simulink library "guidanceLawPathFollowingController"  (R2020a)
settings: Solver=VariableStepAuto  StartTime=0.0  StopTime=10.0  RelTol=1e-3
undefined symbols (not defined in the file or in its folder): env, initializeBussesFromBlock, maxRoll, vhcl
libraries: calculate_vector_magnitude x4, calcFluidDynamicLoads x1, eulAng2RotMat_ul x1, setpointToOutput_cl x1, alphaBeta_ul x1, calc_path_coordinates x1, ctrlAllocMatrix_cl x1, filteredPIDController_ul x1, findClosestPointOnPath x1, findTargetPathParameter x1, gnd2TanRotation_ul x1, spoolingController_cl x1
settings Model: Creator=Ayaz  LastModifiedBy=Ayaz

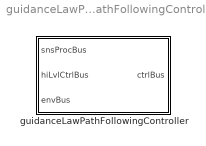
== system guidanceLawPathFollowingController ==
  guidanceLawPathFollowingController : Subsystem  LoadFcn=initializeBussesFromBlock(gcb)  InitFcn=initializeBussesFromBlock(gcb)  StartFcn=initializeBussesFromBlock(gcb)  mask{pathCtrl=90, vcl=vhcl, en=env}
      mask prompts: pathCtrl "Controller object"; vcl "Vehicle object"; en "Environment object"
      mask DialogControl ParameterGroupVar Prompt: Controller parameters
      mask DialogControl Container3 Prompt: Vehicle parameters
      mask DialogControl Container4 Prompt: Environment parameter

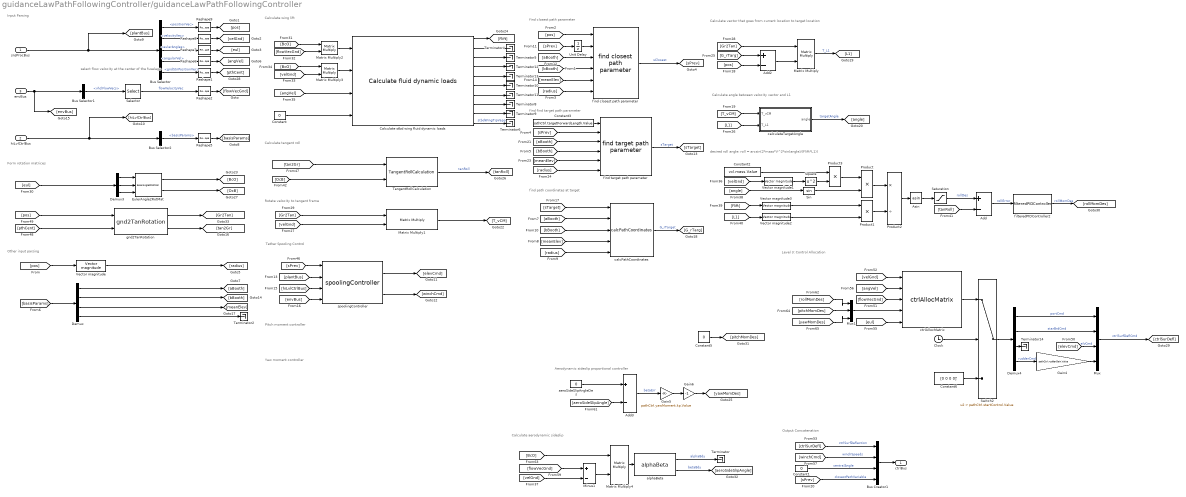
== system guidanceLawPathFollowingController/guidanceLawPathFollowingController ==
  note: Other input parsing
  note: Form rotation matrices
  note: Calculate wing lift
  note: Rotate velocity to tangent frame
  note: select flow velocity at the center of the fuselage
  note: Tether Spooling Control
  note: Input Parsing
  note: find closest path parameter
  note: find find target path parameter
  note: find path coordinates at target
  note: Calculate vector that goes from current location to target location
  note: Calculate angle between velocity vector and L1
  note: desired roll angle: roll = arcsin(2*mass*V^2*sin(angle)/(Flift*L1))
  note: Calculate tangent roll
  note: Output Concatenation
  note: Level 3: Control Allocation
  note: Pitch moment controller
  note: Aerodynamic sideslip proportional controller
  note: Yaw moment controller
  note: Calculate aerodynamic sideslip
  snsProcBus : Inport  OutDataTypeStr=Bus: sensorsProcessingBus
  hiLvlCtrlBus : Inport  Port=2  OutDataTypeStr=Bus: hiLvlCtrlBus
  envBus : Inport  Port=3  OutDataTypeStr=Bus: envBus
  Add : Sum  Inputs=+-
  Add2 : Sum  Inputs=+-
  Add3 : Sum  Inputs=+-
  Asin : Trigonometry  Operator=asin
  Bus Creator1 : BusCreator  Inputs=4  OutDataTypeStr=Bus: fltCtrlBus
      settings: InheritFromInputs=off
  Bus Selector : BusSelector  OutputSignals=positionVec,velocityVec,eulerAngles,angularVel,gndStnPositionVec
  Bus Selector1 : BusSelector  OutputSignals=vhclFlowVecs
  Bus Selector2 : BusSelector  OutputSignals=basisParams
  Calculate stbd wing fluid dynamic loads : calcFluidDynamicLoads/Calculate fluid dynamic loads  aSurf=vcl.stbdWing  sRef=vhcl.fluidRefArea.Value  rArm_LE=vcl.fluidMomentArms.Value(:,1).*[1;0;1]  rTip_LE=[0;0;0]  fluidDensity=en.water.density.Value
  Clock : Clock
  Constant : Constant  Value=0
  Constant1 : Constant  Value=0
  Constant2 : Constant  Value=vcl.mass.Value  VectorParams1D=off
  Constant3 : Constant  Value=pathCtrl.targetForwardLength.Value  VectorParams1D=off
  Constant5 : Constant  Value=0
  Constant6 : Constant  Value=[0 0 0 0]'
  Demux : Demux
  Demux3 : Demux  Outputs=3
  Demux4 : Demux
  EulerAngle2RotMat : eulAng2RotMat_ul/EulerAngle2RotMat  SystemSampleTime=-1  Latency=0  AutoFrameSizeCalculation=off
  Gain4 : Gain  Gain=pathCtrl.rudderGain.Value
  Gain5 : Gain  Gain=pathCtrl.yawMoment.kp.Value
  Gain6 : Gain  Gain=-1
  Matrix Multiply{,1..4} (5 alike) : Product  Multiplication=Matrix(*)
  Minus1 : Sum  Inputs=+-
  Mux : Mux
  Mux1 : Mux  Inputs=3
  Product : Product
  Product1 : Product
  Product2 : Product  Inputs=*/
  Product3 : Product
  Reshape{1..2,5..9} (7 alike) : Reshape  OutputDimensionality=Column vector (2-D)
  Saturation : Saturate  UpperLimit=maxRoll*pi/180  LowerLimit=-maxRoll*pi/180
  Selector : Selector  NumberOfDimensions=2  InputPortWidth=3  IndexOptions=Select all,Index vector (dialog)  Indices=[1 3],5  OutputSizes=1,1
  Sin : Trigonometry
  Square : Math  Operator=square  SaturateOnIntegerOverflow=on
  Switch2 : Switch  Criteria=u2 > Threshold  Threshold=pathCtrl.startControl.Value
  TangentRollCalculation : setpointToOutput_cl/desiredMoment/TangentRollCalculation  SystemSampleTime=-1  Latency=0  AutoFrameSizeCalculation=off
  Terminator{,2,4..6,8..14} (12 alike) : Terminator
  Unit Delay : UnitDelay  SampleTime=-1  HasFrameUpgradeWarning=on
  Vector magnitude{,1..3} (4 alike) : calculate_vector_magnitude/Vector magnitude  SystemSampleTime=-1  Latency=0  AutoFrameSizeCalculation=off
  aeroSideSlipAngleDes : Constant  Value=0
  alphaBeta : alphaBeta_ul/alphaBeta  SystemSampleTime=-1  Latency=0  AutoFrameSizeCalculation=off
  calcPathCoordinates : calc_path_coordinates/calcPathCoordinates  SystemSampleTime=-1  Latency=0  AutoFrameSizeCalculation=off
  calculateTargetAngle : Subsystem
  ctrlAllocMatrix : ctrlAllocMatrix_cl/ctrlAllocMatrix  aeroStruct=vcl.struct('OCT.aeroSurf')  fluidDensity=en.water.density.Value
  filteredPIDController2 : filteredPIDController_ul/filteredPIDController  kp=pathCtrl.rollMoment.kp.Value  ki=0  kd=pathCtrl.rollMoment.kd.Value  Value=pathCtrl.rollMoment.tau.Value  externalReset=none
  find closest path parameter : findClosestPointOnPath/find closest path parameter  maxBackward=0  maxForward=0.25  tau=0.618  convergeTol=1e-4  MaxIters=25
  find target path parameter : findTargetPathParameter/find target path parameter  maxBackward=0  maxForward=0.25  tau=0.618  convergeTol=1e-4  MaxIters=25
  gnd2TanRotation : gnd2TanRotation_ul/gnd2TanRotation  SystemSampleTime=-1  Latency=0  AutoFrameSizeCalculation=off
  spoolingController : spoolingController_cl/spoolingController  SystemSampleTime=-1  Latency=0  AutoFrameSizeCalculation=off
  ctrlBus : Outport  OutDataTypeStr=Bus: fltCtrlBus  VectorParamsAs1DForOutWhenUnconnected=off
  wires:
  Bus Selector/1 -> Reshape9/1  "<positionVec>"
  Bus Selector/2 -> Reshape8/1  "<velocityVec>"
  hiLvlCtrlBus/1 -> Bus Selector2/1, [hiLvlCtrlBus]
  Reshape8/1 -> [velGnd]
  snsProcBus/1 -> Bus Selector/1, [plantBus]
  Bus Selector/4 -> Reshape6/1  "<angularVel>"
  Reshape9/1 -> [pos]
  Reshape6/1 -> [angVel]
  Bus Selector2/1 -> Reshape5/1  "<basisParams>"
  Reshape7/1 -> [eul]
  Selector/1 -> Reshape2/1  "flowVelocityVec"
  Bus Selector/3 -> Reshape7/1  "<eulerAngles>"
  Reshape5/1 -> [basisParams]
  Reshape1/1 -> [pthCent]
  Bus Selector/5 -> Reshape1/1  "<gndStnPositionVec>"
  Bus Selector1/1 -> Selector/1  "<vhclFlowVecs>"
  envBus/1 -> [envBus], Bus Selector1/1
  Reshape2/1 -> [flowVecGnd]
  [plantBus] -> spoolingController/2
  spoolingController/1 -> [elevCmd]
  [sPrev] -> spoolingController/1
  spoolingController/2 -> [winchCmd]
  [envBus] -> spoolingController/4
  [hiLvlCtrlBus] -> spoolingController/3
  find closest path parameter/1 -> [sPrev]  "sClosest"
  [bBooth] -> find closest path parameter/4
  Unit Delay/1 -> find closest path parameter/2
  [aBooth] -> find closest path parameter/3
  [sPrev] -> Unit Delay/1
  [pos] -> find closest path parameter/1
  [meanElev] -> find closest path parameter/5
  [radius] -> find closest path parameter/6
  Vector magnitude/1 -> [radius]
  [sPrev] -> find target path parameter/2
  [aBooth] -> find target path parameter/3
  find target path parameter/1 -> [sTarget]  "sTarget"
  [meanElev] -> find target path parameter/5
  [radius] -> find target path parameter/6
  Constant3/1 -> find target path parameter/1
  [bBooth] -> find target path parameter/4
  Demux/1 -> [aBooth]
  Demux/2 -> [bBooth]
  Demux/3 -> [meanElev]
  [basisParams] -> Demux/1
  Demux/4 -> Terminator2/1
  [aBooth] -> calcPathCoordinates/2
  [bBooth] -> calcPathCoordinates/3
  [radius] -> calcPathCoordinates/5
  [meanElev] -> calcPathCoordinates/4
  [sTarget] -> calcPathCoordinates/1
  calcPathCoordinates/1 -> [G_rTarg]  "G_rTarget"
  [pos] -> Vector magnitude/1
  Add2/1 -> Matrix Multiply/2
  [G_rTarg] -> Add2/1
  [pos] -> Add2/2
  Matrix Multiply/1 -> [L1]  "T_L1"
  [T_vCM] -> calculateTargetAngle/1(T_vCM)
  [Gr2Tan] -> Matrix Multiply/1
  [Gr2Tan] -> Matrix Multiply1/1
  [velGnd] -> Matrix Multiply1/2
  Matrix Multiply1/1 -> [T_vCM]
  Demux3/1 -> EulerAngle2RotMat/1
  Demux3/2 -> EulerAngle2RotMat/2
  Demux3/3 -> EulerAngle2RotMat/3
  [eul] -> Demux3/1
  EulerAngle2RotMat/1 -> [BcO]
  EulerAngle2RotMat/2 -> [OcB]
  Matrix Multiply2/1 -> Calculate stbd wing fluid dynamic loads/1
  [BcO] -> Matrix Multiply2/1
  [flowVecGnd] -> Matrix Multiply2/2
  Matrix Multiply3/1 -> Calculate stbd wing fluid dynamic loads/2
  [BcO] -> Matrix Multiply3/1
  [velGnd] -> Matrix Multiply3/2
  [angVel] -> Calculate stbd wing fluid dynamic loads/3
  Constant/1 -> Calculate stbd wing fluid dynamic loads/4
  Calculate stbd wing fluid dynamic loads/1 -> [Flift]
  Calculate stbd wing fluid dynamic loads/2 -> Terminator4/1
  Calculate stbd wing fluid dynamic loads/3 -> Terminator5/1
  Calculate stbd wing fluid dynamic loads/9 -> Terminator9/1
  Calculate stbd wing fluid dynamic loads/8 -> Terminator8/1
  Calculate stbd wing fluid dynamic loads/7 -> Terminator11/1
  Calculate stbd wing fluid dynamic loads/6 -> Terminator10/1
  Calculate stbd wing fluid dynamic loads/5 -> Terminator13/1
  Calculate stbd wing fluid dynamic loads/4 -> Terminator12/1
  Calculate stbd wing fluid dynamic loads/10 -> Terminator6/1  "stbdWingTipVapp"
  Product3/1 -> Product/1
  [Flift] -> Vector magnitude3/1
  Product1/1 -> Product2/2
  Product2/1 -> Asin/1
  [L1] -> Vector magnitude2/1
  Vector magnitude2/1 -> Product1/2
  Sin/1 -> Product/2
  [angle] -> Sin/1
  Product/1 -> Product2/1
  Vector magnitude1/1 -> Square/1
  [velGnd] -> Vector magnitude1/1
  [OcB] -> TangentRollCalculation/2
  TangentRollCalculation/1 -> [tanRoll]  "tanRoll"
  [tan2Gr] -> TangentRollCalculation/1
  Square/1 -> Product3/2
  Constant2/1 -> Product3/1
  Vector magnitude3/1 -> Product1/1
  Asin/1 -> Saturation/1
  [pos] -> gnd2TanRotation/1
  [pthCent] -> gnd2TanRotation/2
  gnd2TanRotation/1 -> [Gr2Tan]
  gnd2TanRotation/2 -> [tan2Gr]
  Saturation/1 -> Add/1  "rollDes"
  ctrlAllocMatrix/1 -> Switch2/1
  Demux4/4 -> Gain4/1  "rudderCmd"
  [angVel] -> ctrlAllocMatrix/2
  Demux4/3 -> Terminator14/1
  Demux4/1 -> Mux/1  "portCmd"
  Mux1/1 -> ctrlAllocMatrix/4
  Clock/1 -> Switch2/2
  Gain4/1 -> Mux/4
  [eul] -> ctrlAllocMatrix/5
  [elevCmd] -> Mux/3  "elvCmd"
  [winchCmd] -> Bus Creator1/2  "winchSpeeds"
  [flowVecGnd] -> ctrlAllocMatrix/3
  Switch2/1 -> Demux4/1
  [velGnd] -> ctrlAllocMatrix/1
  [sPrev] -> Bus Creator1/4  "closestPathVariable"
  Demux4/2 -> Mux/2  "starBrdCmd"
  Mux/1 -> [ctrlSurDefl]  "ctrlSurfDeflCmd"
  Bus Creator1/1 -> ctrlBus/1
  [ctrlSurDefl] -> Bus Creator1/1  "ctrlSurfDeflection"
  Constant6/1 -> Switch2/3
  Constant1/1 -> Bus Creator1/3  "centralAngle"
  filteredPIDController2/1 -> [rollMomDes]  "rollMomDes"
  Add3/1 -> Gain5/1  "betaErr"
  [BcO] -> Matrix Multiply4/1
  Gain5/1 -> Gain6/1
  [flowVecGnd] -> Minus1/1
  [aeroSideSlipAngle] -> Add3/2
  Matrix Multiply4/1 -> alphaBeta/1
  Minus1/1 -> Matrix Multiply4/2
  Gain6/1 -> [yawMomDes]
  [velGnd] -> Minus1/2
  aeroSideSlipAngleDes/1 -> Add3/1
  alphaBeta/2 -> [aeroSideSlipAngle]  "betaBdy"
  alphaBeta/1 -> Terminator/1  "alphaBdy"
  Constant5/1 -> [pitchMomDes]
  [rollMomDes] -> Mux1/1
  [pitchMomDes] -> Mux1/2
  [yawMomDes] -> Mux1/3
  [tanRoll] -> Add/2
  [L1] -> calculateTargetAngle/2(T_L1)
  calculateTargetAngle/1(angle) -> [angle]  "targetAngle"
  Add/1 -> filteredPIDController2/1  "rollError"

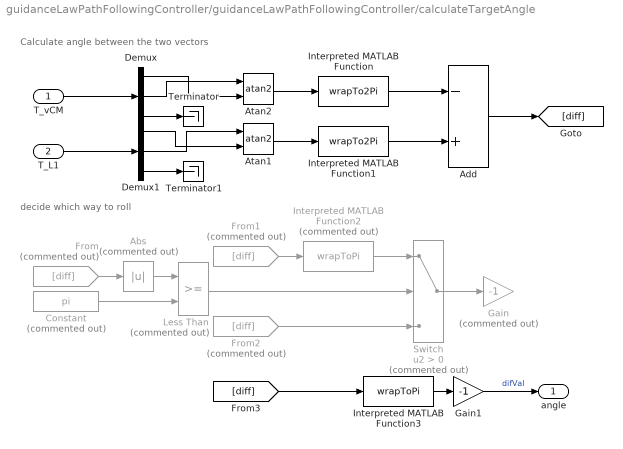
== system guidanceLawPathFollowingController/guidanceLawPathFollowingController/calculateTargetAngle ==
  note: Calculate angle between the two vectors
  note: decide which way to roll
  T_vCM : Inport
  T_L1 : Inport  Port=2
  Abs : Abs  Commented=on
  Add : Sum  Inputs=-+
  Atan1 : Trigonometry  Operator=atan2
  Atan2 : Trigonometry  Operator=atan2
  Constant : Constant  Commented=on  Value=pi
  Demux : Demux  Outputs=3
  Demux1 : Demux  Outputs=3
  From : From  Commented=on  GotoTag=diff
  From1 : From  Commented=on  GotoTag=diff
  From2 : From  Commented=on  GotoTag=diff
  Gain : Gain  Commented=on  Gain=-1
  Gain1 : Gain  Gain=-1
  Interpreted MATLAB Function : MATLABFcn  MATLABFcn=wrapTo2Pi
  Interpreted MATLAB Function1 : MATLABFcn  MATLABFcn=wrapTo2Pi
  Interpreted MATLAB Function2 : MATLABFcn  Commented=on  MATLABFcn=wrapToPi
  Interpreted MATLAB Function3 : MATLABFcn  MATLABFcn=wrapToPi
  Less Than : RelationalOperator  Commented=on  OutDataTypeStr=boolean  RndMeth=Simplest
  Switch : Switch  Commented=on  Criteria=u2 > Threshold
  Terminator : Terminator
  Terminator1 : Terminator
  angle : Outport
  wires:
  Interpreted MATLAB Function/1 -> Add/1
  T_vCM/1 -> Demux/1
  Atan2/1 -> Interpreted MATLAB Function/1
  Less Than/1 -> Switch/2
  T_L1/1 -> Demux1/1
  Constant/1 -> Less Than/2
  Demux/1 -> Atan2/2
  Atan1/1 -> Interpreted MATLAB Function1/1
  Demux1/1 -> Atan1/2
  Add/1 -> [diff]
  Interpreted MATLAB Function1/1 -> Add/2
  Demux/3 -> Terminator/1
  Demux1/3 -> Terminator1/1
  Switch/1 -> Gain/1
  Demux1/2 -> Atan1/1
  Demux/2 -> Atan2/1
  From/1 -> Abs/1
  From2/1 -> Switch/3
  Interpreted MATLAB Function2/1 -> Switch/1
  From1/1 -> Interpreted MATLAB Function2/1
  Abs/1 -> Less Than/1
  [diff] -> Interpreted MATLAB Function3/1
  Interpreted MATLAB Function3/1 -> Gain1/1
  Gain1/1 -> angle/1  "difVal"
